simulink model "ShanthanECE229HW3Sim"  (R2024b)
settings: Solver=VariableStepAuto  StartTime=0.0  StopTime=T  MaxStep=MaxStep  RelTol=RelTol
InitFcn:
  | ShanthanHW3ECE229InitScript
values from neighbouring files (symbols this model uses):
  J = 10    [ShanthanHW3ECE229InitScript.m]
  parameters = struct()    [ShanthanHW3ECE229InitScript.m]
  T = 50    [ShanthanHW3ECE229InitScript.m]
  x0 = [-0.6536;-0.7568;0;2]    [ShanthanHW3ECE229InitScript.m]
libraries: HyEQ_Library x1
settings Model: Creator=heeirthan  LastModifiedBy=heeirthan

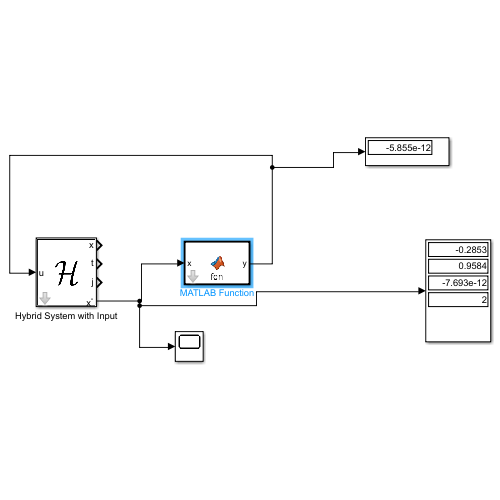
[thumbnail: Simulink's stored preview of the top-level diagram]
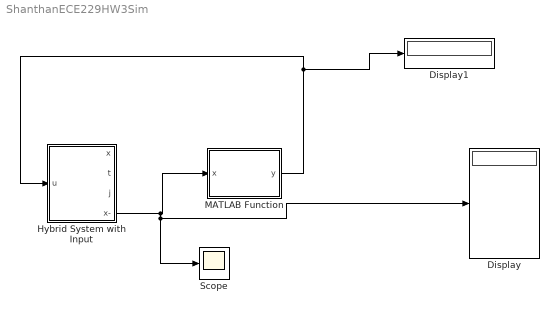
== system ShanthanECE229HW3Sim ==
  Display : Display
  Display1 : Display
  Hybrid System with Input : Subsystem  LoadFcn=set_param(gcb,'LinkStatus','none')  mask(Hybrid System with Inputs){x0=x0, input_dim=1, parameters=parameters, T=T, J=J, rule=Jump}
      mask prompts: x0 "Initial Condition (column vector)"; input_dim "Input Dimension (positive integer)"; T "Flow Horizon (nonnegative real)"; J "Jump Horizon (nonnegative integer)"; rule "Flow/Jump Priorty Rule"
      mask help:
      | To modify (f, g, C, D) for this block, "Look inside" the block mask by either clicking the down arrow in the lower-left corner or selecting "Mask" > "Look Under Mask" from the context menu.
      |
      | For instructions how to use this block, see the
      mask init:
      | state_dim = numel(x0);
      settings: CopyFcn=|
      | set_param(gcb,'LinkStatus','none'),
      | set_param(gcs, 'MaxStep', 'MaxStep', 'RelTol', 'RelTol','StopTime', 'T')
      mask Help:
      | To modify (f, g, C, D) for this block, "Look inside" the block mask by either clicking the down arrow in the lower-left corner or selecting "Mask" > "Look Under Mask" from the context menu.
      | 
      | The value given in the 'parameters' field is passed as the last input argument for f, g, C, and D. Any MATLAB object can be used, but we recommend using a struct. For example, in the initialization script, a parameters struct can be defined as followed.
      |   parameters = struct();
      |   parameters.A = eye(2);
      |   parameters.B = [1; 0];
      | 
      | The output "x-" is the state output delayed by one integration step. Use this output to break algebraic loops.
      mask TypeOptions x0: Integrator System/x0
      mask TypeOptions T: Integrator System/T
      mask TypeOptions J: Integrator System/J
      mask TypeOptions rule: Jump | Flow | Random
      mask DialogControl Control2 Prompt: Introduction to the HyEQ Simulink-based Library
      mask DialogControl Control2 Callback: hybrid.internal.openHelp('Help_SimulinkLibrary')
      mask DialogControl Container3 Prompt: System Configuration
      mask DialogControl Container2 Prompt: Solver Options
      mask Display:
      | image('Hcal.jpg')
      | port_label('output', 1, 'x')
      | port_label('output', 2, 't')
      | port_label('output', 3, 'j')
      | port_label('output', 4, 'x^-','texmode', 'on')
      | port_label('input', 1, 'u')
  MATLAB Function : MATLAB Function  TreatAsAtomicUnit=on
  Scope : Scope
  wires:
  MATLAB Function/1(y) -> Display1/1, Hybrid System with Input/1(u)
  Hybrid System with Input/4(x-) -> Display/1, Scope/1, MATLAB Function/1(x)

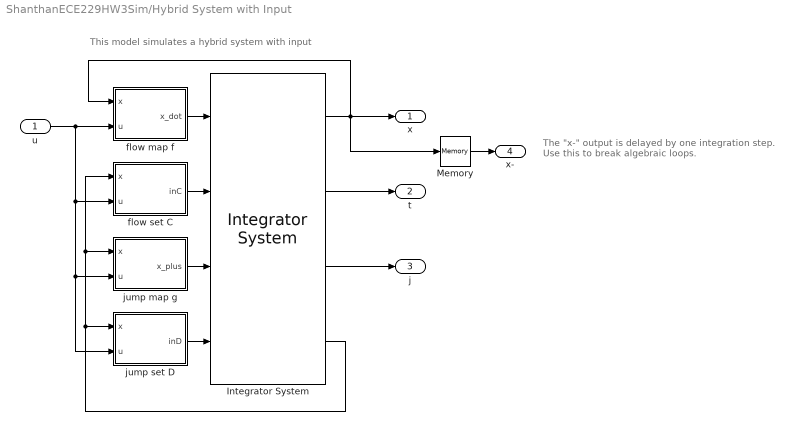
== system ShanthanECE229HW3Sim/Hybrid System with Input ==
  note: This model simulates a hybrid system with input
  note: The "x-" output is delayed by one integration step. Use this to break algebraic loops.
  u : Inport  PortDimensions=input_dim
  Integrator System : HyEQ_Library/Other/Integrator System  Priority=2  T=T  J=J  x0=x0  rule=rule
      settings: SourceProductName=Hybrid Equations Toolbox
  Memory : Memory  InitialCondition=x0
  flow map f : MATLAB Function  TreatAsAtomicUnit=on
  flow set C : MATLAB Function  TreatAsAtomicUnit=on
  jump map g : MATLAB Function  TreatAsAtomicUnit=on
  jump set D : MATLAB Function  TreatAsAtomicUnit=on
  x : Outport  PortDimensions=state_dim
  t : Outport  Port=2  PortDimensions=1
  j : Outport  Port=3  PortDimensions=1
  x- : Outport  Port=4  PortDimensions=state_dim
  wires:
  Memory/1 -> x-/1
  jump map g/1(x_plus) -> Integrator System/3
  jump set D/1(inD) -> Integrator System/4
  u/1 -> jump set D/2(u), jump map g/2(u), flow set C/2(u), flow map f/2(u)
  Integrator System/3 -> j/1
  Integrator System/2 -> t/1
  flow set C/1(inC) -> Integrator System/2
  Integrator System/1 -> x/1, flow map f/1(x), Memory/1
  Integrator System/4 -> jump map g/1(x), flow set C/1(x), jump set D/1(x)
  flow map f/1(x_dot) -> Integrator System/1

== matlab function ShanthanECE229HW3Sim/Hybrid System with Input/flow map f ==
  data: x input size=state_dim; u input size=input_dim; x_dot output size=state_dim; parameters parameter
function x_dot = f(x, u, parameters)
   % Define flow map here.
   a = parameters; 
   x_dot = [-x(2)*x(3);x(1)*x(3);u;0];
end

== matlab function ShanthanECE229HW3Sim/Hybrid System with Input/flow set C ==
  data: x input size=state_dim; u input size=input_dim; inC output size=1; parameters parameter
function inC = C(x, u, parameters)
   % Define flow set indictor function here.
   k1 = parameters.k1;
   k2 = parameters.k2;
   delta = parameters.delta;
   V1 = 0.5 - 0.5*cos((k1/2)*(1-x(1)))*x(1) + 0.5*sin((k1/2)*(1-x(1)))*x(2);
   V2 = 0.5 - 0.5*cos((k2/2)*(1-x(1)))*x(1) + 0.5*sin((k2/2)*(1-x(1)))*x(2);
   V = [V1;V2];
   M = min(V(1),V(2));

    
   inC = M - V(round(x(4))) >= -delta;
end

== matlab function ShanthanECE229HW3Sim/Hybrid System with Input/jump map g ==
  data: x input size=state_dim; u input size=input_dim; x_plus output size=state_dim; parameters parameter
function x_plus = g(x, u, parameters)
   if x(4) == 1
     q = 2;
   else
     q = 1;
   end    
   x_plus = [x(1);x(2);x(3);q];
end

== matlab function ShanthanECE229HW3Sim/Hybrid System with Input/jump set D ==
  data: x input size=state_dim; u input size=input_dim; inD output size=1; parameters parameter
function inD = D(x, u, parameters)
   % Define jump set indicator function here.
   k1 = parameters.k1;
   k2 = parameters.k2;
   delta = parameters.delta;
   V1 = 0.5 - 0.5*cos((k1/2)*(1-x(1)))*x(1) + 0.5*sin((k1/2)*(1-x(1)))*x(2);
   V2 = 0.5 - 0.5*cos((k2/2)*(1-x(1)))*x(1) + 0.5*sin((k2/2)*(1-x(1)))*x(2);
   V = [V1;V2];
   M = min(V(1),V(2));

    
   inD = M - V(round(x(4))) <= -delta;
end

== matlab function ShanthanECE229HW3Sim/MATLAB Function ==
  data: x input; y output
function y = fcn(x)
   k1 = 1.5;
   k2 = -1.5;
   grad_V1 = 0.25*(k1*x(2) + 2)*(x(2)*cos(0.5*k1*(x(1) - 1)) - x(1)*sin(0.5*k1*(x(1) - 1)));
   grad_V2 = 0.25*(k2*x(2) + 2)*(x(2)*cos(0.5*k2*(x(1) - 1)) - x(1)*sin(0.5*k2*(x(1) - 1)));
   grad_V = [grad_V1;grad_V2];

y = -grad_V(round(x(4)))-x(3);
